simulink model "Electrical_System_2018b_obfs"  (R2019b)
settings: Solver=VariableStepAuto  StartTime=0.0  StopTime=5  RelTol=1e-3  AbsTol=1e-3  EnableMultiTasking=on
InitFcn:
  | Steady_State_Initialisation;
StopFcn:
  | %sscexplore(simlog);
  | %Logging
undefined symbols (not defined in the file): abrlhklxvp, aexgmhuedq, afmfmjnutg, afpphrjpnc, ahuxbyvruc, alarvljztt, amxnyqmnuw, aodrlwvqie, aolhmuplyq, aqpmguuqkg, auesgwirzl, aurophlnng, awamelrhru, ayfhvxflxn, azxkacuhqc, babszerikg, bawhdqanwq, bevoqecvei, bltjvqbchx, bmqsuewujl, bsmyqjfgnf, btvjbsmnve, bywgxqeadw, bziaduxaer, bzmcmdqocb, bzsvyvetat, ccsjnrbsih, cdvenygxwh, cedkrnslhx, cjheorclzs, cjrdshrtqx, ckhavyhcza, ckxewznhlz, cmrcgyiplk, conenicnws, cqkejbgjnn, csfnuwymhe, cunupkhwbh, cwzfvzuxxh, dcadmadufn, dcfponivnv, ddtrqjrhjn, dfhoxvkqas, dfrhtcwpne, dfvomcagjv, djijwylxea, dnmeqksrrm, dnzewbdkaa, dsqcykyxav, dtswwlttmm, ecumpidjtv, edegaywrct, ejjjsmnejc, eknqnehjdz, emvdetzouf, esxbqkbahr, etnkkbreiq, eunoiiiirw, ewewcuedir, fatkfxdhtc ... (+386)
libraries: fl_lib x802, ee_lib x362, fl_ps_legacy_lib x160, nesl_utility x85
(part 11 of 26)

== system Electrical_System_2018b_obfs/Redacted_1221/Redacted_7996/Redacted_1/Redacted_4377/Redacted_6082/Redacted_4288 ==
  Redacted_1420 : ee_lib/Passive/Thermal/Thermal Resistor  R=csfnuwymhe K/W  T_specify=off  T_priority=None  T=dfrhtcwpne K  T_nominal_specify=off  T_nominal_unit=K  T_nominal_value=undcbzrngw  Q_specify=off  Q_priority=None  Q=qyyvrynvtf W  Q_nominal_specify=off  Q_nominal_unit=W  Q_nominal_value=fykywgxewt
      settings: SourceProductName=Simscape Electrical  SourceProductBaseCode=PS  InternalSimscapePortConfiguration="{\"Bottom\":[],\"Left\":[{\"id\":\"A\",\"label\":\"A\",\"type\":\"foundation.thermal.thermal\"}],\"Right\":[{\"id\":\"B\",\"label\":\"B\",\"type\":\"foundation.thermal.thermal\"}],\"Top\":[]}"
  Redacted_3053 : ee_lib/Passive/Thermal/Thermal Resistor  R=feuklzgtpa K/W  T_specify=off  T_priority=None  T=qwktvjvfys K  T_nominal_specify=off  T_nominal_unit=K  T_nominal_value=arolkdlhmd  Q_specify=off  Q_priority=None  Q=djhelqxest W  Q_nominal_specify=off  Q_nominal_unit=W  Q_nominal_value=dkqmeratgj
      settings: SourceProductName=Simscape Electrical  SourceProductBaseCode=PS  InternalSimscapePortConfiguration="{\"Bottom\":[],\"Left\":[{\"id\":\"A\",\"label\":\"A\",\"type\":\"foundation.thermal.thermal\"}],\"Right\":[{\"id\":\"B\",\"label\":\"B\",\"type\":\"foundation.thermal.thermal\"}],\"Top\":[]}"
  Redacted_5187 : fl_lib/Electrical/Electrical Elements/Switch  R_closed=iidrcmgruo Ohm  G_open=cwflxapbrg 1/Ohm  Threshold=wtaszsnldr  i_specify=off  i_priority=None  i=cfjwrmlajq A  i_nominal_specify=off  i_nominal_unit=A  i_nominal_value=qzidrdxbsm  v_specify=off  v_priority=None  v=hrbzqwpexo V  v_nominal_specify=off  v_nominal_unit=V  v_nominal_value=oarcvjnccc
      settings: SourceProductName=Simscape
  Redacted_5716 : fl_lib/Electrical/Electrical Elements/Switch  R_closed=krkbgwsxlo Ohm  G_open=nwjalbnmwo 1/Ohm  Threshold=wlnjmfizfx  i_specify=off  i_priority=None  i=xtkvqzsayg A  i_nominal_specify=off  i_nominal_unit=A  i_nominal_value=nzimhpxyaj  v_specify=off  v_priority=None  v=dcozybqfae V  v_nominal_specify=off  v_nominal_unit=V  v_nominal_value=cwsubwwopk
      settings: SourceProductName=Simscape
  Redacted_631 : ee_lib/Semiconductors & Converters/Diode  ModelType=kwymznercn  Vf=bzeobnkmpp V  Ron=ogzcuqezum Ohm  Goff=hboakganul S  prmExp=tspwxvmtix  I12=vzhmfidnsx A  V12=lzcdoaedsk V  IS=lxuhqgdzyf A  ec=lgmvvpmtfb  I1=wubgixerlf A  V1=ghqnutyshn V  RS=yfueffmaxl Ohm  Tmeas=ydajfmxqbx degC  N_series=yivbhcvoir  N_parallel=htzntkphxa  Rz=qvvvhxwbpi Ohm  BV=ymjzdmieqs V  C_param=msvgljfcfw  CJ=zsrrieohii pF  CJ0=tuthjrqdnh pF  VJ=nycerhqgyj V  Mgrad=qvizemveid  Vvec=qlenbgnmqk V  Cvec=bligwbbtgp pF  FC=roozurrocc  Q_param=xkglsmbrbh  iRM=qahgubavsm A  iF=pufyexdedl A  didt=isjydruslg A/us  trr_factor=dffqwpsdyp  trr=anfkerbzue ns  Qrr=deomtvnwwe s*uA  TT=lrekwszonl ns  tau=iyastrgkxi ns  T_param=kjwuhembzs  IS_T2=mmckjlxiwy A  I1_T2=llsygjllnm A  V1_T2=ebzpqvnskm V  Tmeas2=dgihdwdint degC  EG_param=vfglbqzjmq  EG=vnjpxdvxmw eV  XTI_param=uocmdbuhnh  XTI=mybmalgdic  dBVdT=fpdhcmbsix V/K  Tdevice=fyegxrufcw degC  i_specify=off  i_priority=None  i=lkokslneyy A  i_nominal_specify=off  i_nominal_unit=A  i_nominal_value=hoeahmmfuu  v_specify=off  v_priority=None  v=jwstxjltpj V  v_nominal_specify=off  v_nominal_unit=V  v_nominal_value=vzfhxnllbc  i_capacitor_specify=off  i_capacitor_priority=None  i_capacitor=myvfxzqlck A  i_capacitor_nominal_specify=off  i_capacitor_nominal_unit=A  i_capacitor_nominal_value=roqvolylnm  v_capacitor_specify=off  v_capacitor_priority=None  v_capacitor=gptluhsrhz V  v_capacitor_nominal_specify=off  v_capacitor_nominal_unit=V  v_capacitor_nominal_value=alzbeepcwm  power_dissipated_specify=off  power_dissipated_priority=None  power_dissipated=uijibnuhos W  power_dissipated_nominal_specify=off  power_dissipated_nominal_unit=W  power_dissipated_nominal_value=lbddeeurpg  thermal_network_parameterization=frunhdzzzq  Rth=ipffswvaig K/W  Rth_Foster=tpgcjeuyzq K/W  thermal_mass_parameterization=jwlodfpkvm  thermal_mass=ehnyrrnqzl J/K  thermal_mass_Foster=unmbisyvtm J/K  thermal_time_constant=oypiywoukf s  thermal_time_constant_Foster=xnmvgxpcww s  thermal_mass_initial_temperatures=zwgjhousxc degC
      settings: SourceProductName=Simscape Electrical  InternalSimscapePortConfiguration="{\"Bottom\":[],\"Left\":[{\"id\":\"p\",\"label\":\"\",\"type\":\"foundation.electrical.electrical\"},{\"id\":\"H\",\"label\":\"H\",\"type\":\"foundation.thermal.thermal\"}],\"Right\":[{\"id\":\"n\",\"label\":\"\",\"type\":\"foundation.electrical.electrical\"}],\"Top\":[]}"
  Redacted_6763 : ee_lib/Semiconductors & Converters/Diode  ModelType=clgixcnwoc  Vf=ftpzcjmppy V  Ron=dbcidwevvn Ohm  Goff=yhrmcwzgue S  prmExp=aisizesfzq  I12=lacnnvocyc A  V12=pbpbsjubgs V  IS=xamdbquppu A  ec=eeecjfdprz  I1=yjljdcozpv A  V1=ffbopghzjw V  RS=wcqnbvzzev Ohm  Tmeas=kbuiibngbo degC  N_series=qqlilfwukw  N_parallel=fxbsiddyro  Rz=dodwndnmkr Ohm  BV=liehghwjmv V  C_param=vktsvahwle  CJ=fhntaxxfft pF  CJ0=qumaznckyu pF  VJ=xpoblmifuo V  Mgrad=ocusdggsnv  Vvec=seffqhedpz V  Cvec=ohcmggolrz pF  FC=yxsxrkinug  Q_param=bvzohlmuww  iRM=xicczpmsfr A  iF=rkcnntyhvb A  didt=vtudfiaipt A/us  trr_factor=rqvaooxfvk  trr=tvwihwyihb ns  Qrr=kulozvhoez s*uA  TT=nitkbtqglp ns  tau=ubqxhynwqh ns  T_param=igxsyorppi  IS_T2=mqvbxmpxvg A  I1_T2=armqecybmn A  V1_T2=muvfioogix V  Tmeas2=ppsjgixytg degC  EG_param=xjxvdcpxwh  EG=agihhvisij eV  XTI_param=yuocwdmjkw  XTI=xoszctygzp  dBVdT=uoohrvaigf V/K  Tdevice=qhfnbogqqg degC  i_specify=off  i_priority=None  i=qtedmgmqsm A  i_nominal_specify=off  i_nominal_unit=A  i_nominal_value=mqkthilpvy  v_specify=off  v_priority=None  v=itpbbundcp V  v_nominal_specify=off  v_nominal_unit=V  v_nominal_value=ykhzflpcnx  i_capacitor_specify=off  i_capacitor_priority=None  i_capacitor=uryfeeajta A  i_capacitor_nominal_specify=off  i_capacitor_nominal_unit=A  i_capacitor_nominal_value=ftxeerromd  v_capacitor_specify=off  v_capacitor_priority=None  v_capacitor=hddhodbyvb V  v_capacitor_nominal_specify=off  v_capacitor_nominal_unit=V  v_capacitor_nominal_value=yzdcvmjrfh  power_dissipated_specify=off  power_dissipated_priority=None  power_dissipated=aaxygncreu W  power_dissipated_nominal_specify=off  power_dissipated_nominal_unit=W  power_dissipated_nominal_value=xuxnetzqve  thermal_network_parameterization=zrkkuhurzb  Rth=odsbqwesbo K/W  Rth_Foster=ibbukupzba K/W  thermal_mass_parameterization=laqxzbiuja  thermal_mass=jqetfysksy J/K  thermal_mass_Foster=rleuvpzybd J/K  thermal_time_constant=vfwhldlplc s  thermal_time_constant_Foster=sredobdxmn s  thermal_mass_initial_temperatures=gkskoiqoer degC
      settings: SourceProductName=Simscape Electrical  InternalSimscapePortConfiguration="{\"Bottom\":[],\"Left\":[{\"id\":\"p\",\"label\":\"\",\"type\":\"foundation.electrical.electrical\"},{\"id\":\"H\",\"label\":\"H\",\"type\":\"foundation.thermal.thermal\"}],\"Right\":[{\"id\":\"n\",\"label\":\"\",\"type\":\"foundation.electrical.electrical\"}],\"Top\":[]}"
  Redacted_938 : ee_lib/Passive/Thermal/Thermal Resistor  R=virfgdrnfz K/W  T_specify=off  T_priority=None  T=alarvljztt K  T_nominal_specify=off  T_nominal_unit=K  T_nominal_value=joqgdgroxe  Q_specify=off  Q_priority=None  Q=kaqfzywiqi W  Q_nominal_specify=off  Q_nominal_unit=W  Q_nominal_value=zlmidgadwg
      settings: SourceProductName=Simscape Electrical  SourceProductBaseCode=PS  InternalSimscapePortConfiguration="{\"Bottom\":[],\"Left\":[{\"id\":\"A\",\"label\":\"A\",\"type\":\"foundation.thermal.thermal\"}],\"Right\":[{\"id\":\"B\",\"label\":\"B\",\"type\":\"foundation.thermal.thermal\"}],\"Top\":[]}"
  Redacted_2382 : PMIOPort  Side=Left
  Redacted_435 : PMIOPort  Port=2  Side=Left
  Redacted_3794 : PMIOPort  Port=3  Side=Right
  Redacted_28 : PMIOPort  Port=4  Side=Right
  Redacted_1383 : PMIOPort  Port=5  Side=Left
  Redacted_1778 : PMIOPort  Port=6  Side=Right
  connections:
  Redacted_6763/LConn1 -- Redacted_435/RConn1
  Redacted_6763/RConn1 -- Redacted_5716/LConn1
  Redacted_631/LConn2 -- Redacted_938/LConn1
  Redacted_3794/RConn1 -- Redacted_5187/RConn2
  Redacted_631/LConn1 -- Redacted_5187/LConn1
  Redacted_2382/RConn1 -- Redacted_631/RConn1
  Redacted_3053/RConn1 -- Redacted_1420/LConn1 -- Redacted_938/RConn1
  Redacted_1778/RConn1 -- Redacted_5716/RConn1 -- Redacted_5187/RConn1
  Redacted_28/RConn1 -- Redacted_5716/RConn2
  Redacted_1420/RConn1 -- Redacted_1383/RConn1
  Redacted_6763/LConn2 -- Redacted_3053/LConn1

== system Electrical_System_2018b_obfs/Redacted_1221/Redacted_7996/Redacted_1/Redacted_4377/Redacted_6082/Redacted_4413 ==
  Neutral_Negative : Subsystem  VariantControl=Variant1
  Positive_Neutral : Subsystem  VariantControl=Variant3
  Redacted_6190 : Subsystem  VariantControl=Variant2
  Redacted_9976 : PMIOPort  Side=Left
  Redacted_5180 : PMIOPort  Port=2  Side=Left
  Redacted_6712 : PMIOPort  Port=3  Side=Left
  Redacted_6595 : PMIOPort  Port=4  Side=Right
  Redacted_8408 : PMIOPort  Port=5  Side=Right

== system Electrical_System_2018b_obfs/Redacted_1221/Redacted_7996/Redacted_1/Redacted_4377/Redacted_6082/Redacted_4712 ==
  Redacted_2183 : ee_lib/Passive/Thermal/Thermal Resistor  R=uwrxzutslg K/W  T_specify=off  T_priority=None  T=pajgcmnuxp K  T_nominal_specify=off  T_nominal_unit=K  T_nominal_value=oprwgenfni  Q_specify=off  Q_priority=None  Q=vnctjcpbal W  Q_nominal_specify=off  Q_nominal_unit=W  Q_nominal_value=rnairkbzzr
      settings: SourceProductName=Simscape Electrical  SourceProductBaseCode=PS  InternalSimscapePortConfiguration="{\"Bottom\":[],\"Left\":[{\"id\":\"A\",\"label\":\"A\",\"type\":\"foundation.thermal.thermal\"}],\"Right\":[{\"id\":\"B\",\"label\":\"B\",\"type\":\"foundation.thermal.thermal\"}],\"Top\":[]}"
  Redacted_2562 : fl_lib/Electrical/Electrical Elements/Switch  R_closed=vkroixkmza Ohm  G_open=aclkmnqnqn 1/Ohm  Threshold=mqphwqpqtk  i_specify=off  i_priority=None  i=wqsnzdmaqu A  i_nominal_specify=off  i_nominal_unit=A  i_nominal_value=jdsbnyvvrn  v_specify=off  v_priority=None  v=mtgnvxvoef V  v_nominal_specify=off  v_nominal_unit=V  v_nominal_value=xpdcqtwjkq
      settings: SourceProductName=Simscape
  Redacted_4076 : fl_lib/Electrical/Electrical Elements/Switch  R_closed=njwxpudroe Ohm  G_open=unopnvzees 1/Ohm  Threshold=vnjqsgeems  i_specify=off  i_priority=None  i=tvyggmthfk A  i_nominal_specify=off  i_nominal_unit=A  i_nominal_value=fudhxnvthp  v_specify=off  v_priority=None  v=blecxtmuzk V  v_nominal_specify=off  v_nominal_unit=V  v_nominal_value=mxbomhtqdj
      settings: SourceProductName=Simscape
  Redacted_4934 : ee_lib/Passive/Thermal/Thermal Resistor  R=qtaxfrwwfd K/W  T_specify=off  T_priority=None  T=jbhnvsqxgq K  T_nominal_specify=off  T_nominal_unit=K  T_nominal_value=wqgbotzlrn  Q_specify=off  Q_priority=None  Q=oiubxlneqr W  Q_nominal_specify=off  Q_nominal_unit=W  Q_nominal_value=qhrxutyvpm
      settings: SourceProductName=Simscape Electrical  SourceProductBaseCode=PS  InternalSimscapePortConfiguration="{\"Bottom\":[],\"Left\":[{\"id\":\"A\",\"label\":\"A\",\"type\":\"foundation.thermal.thermal\"}],\"Right\":[{\"id\":\"B\",\"label\":\"B\",\"type\":\"foundation.thermal.thermal\"}],\"Top\":[]}"
  Redacted_6160 : ee_lib/Semiconductors & Converters/Diode  ModelType=wxghzbmewo  Vf=incyrzxxzf V  Ron=bufhejqsgj Ohm  Goff=bzmmwltpda S  prmExp=oyufyuxxul  I12=zqevqndhvr A  V12=ntgabtemlm V  IS=esogqbbpag A  ec=mhmrjglsyl  I1=baysikteys A  V1=jddnlczanv V  RS=xilzloxftw Ohm  Tmeas=hshgidoefp degC  N_series=tvwlqlappu  N_parallel=ynyhscmuqe  Rz=biacdhtehh Ohm  BV=vcztypyixs V  C_param=ymjusrygft  CJ=nzixmodzqw pF  CJ0=rmyzhcbopm pF  VJ=texbhuncud V  Mgrad=tkridumood  Vvec=jbuxjwgifj V  Cvec=yijsdqpcdn pF  FC=joqholwqmr  Q_param=iqextqebao  iRM=oosasuiphy A  iF=aqxfnvhdsh A  didt=iuypvkuhmr A/us  trr_factor=dqnmklrpvy  trr=rwbczlghkl ns  Qrr=ashruozjcw s*uA  TT=bxoqkmimcn ns  tau=upkecktgtn ns  T_param=whgrtbtgkt  IS_T2=ytmdinuaho A  I1_T2=poblvhcxkr A  V1_T2=hnwmatqgpq V  Tmeas2=jrgnekkvfk degC  EG_param=tblraoxtej  EG=timwdxryfu eV  XTI_param=btzoraanbl  XTI=wflfvuhjxp  dBVdT=xvknpvwxts V/K  Tdevice=gmzsticnnk degC  i_specify=off  i_priority=None  i=qefslitdry A  i_nominal_specify=off  i_nominal_unit=A  i_nominal_value=qcpugyhbqw  v_specify=off  v_priority=None  v=gggiokbjmg V  v_nominal_specify=off  v_nominal_unit=V  v_nominal_value=scytvwxumi  i_capacitor_specify=off  i_capacitor_priority=None  i_capacitor=qsjysvanbz A  i_capacitor_nominal_specify=off  i_capacitor_nominal_unit=A  i_capacitor_nominal_value=pewfqtvxxi  v_capacitor_specify=off  v_capacitor_priority=None  v_capacitor=bwoefqwwqs V  v_capacitor_nominal_specify=off  v_capacitor_nominal_unit=V  v_capacitor_nominal_value=mkonfywlen  power_dissipated_specify=off  power_dissipated_priority=None  power_dissipated=xgzyrlewkb W  power_dissipated_nominal_specify=off  power_dissipated_nominal_unit=W  power_dissipated_nominal_value=xaufgjttes  thermal_network_parameterization=rhtfzdpkld  Rth=aqkrjbornc K/W  Rth_Foster=cnqtfsutib K/W  thermal_mass_parameterization=xysbimjfwi  thermal_mass=ujjibidbol J/K  thermal_mass_Foster=dehixscchy J/K  thermal_time_constant=prtxkbhlrj s  thermal_time_constant_Foster=tazbjthomj s  thermal_mass_initial_temperatures=qkntalstxl degC
      settings: SourceProductName=Simscape Electrical  InternalSimscapePortConfiguration="{\"Bottom\":[],\"Left\":[{\"id\":\"p\",\"label\":\"\",\"type\":\"foundation.electrical.electrical\"},{\"id\":\"H\",\"label\":\"H\",\"type\":\"foundation.thermal.thermal\"}],\"Right\":[{\"id\":\"n\",\"label\":\"\",\"type\":\"foundation.electrical.electrical\"}],\"Top\":[]}"
  Redacted_7653 : ee_lib/Passive/Thermal/Thermal Resistor  R=tnulhwbazf K/W  T_specify=off  T_priority=None  T=mbqcmvdwox K  T_nominal_specify=off  T_nominal_unit=K  T_nominal_value=ayrbujabnr  Q_specify=off  Q_priority=None  Q=sfclfeggiu W  Q_nominal_specify=off  Q_nominal_unit=W  Q_nominal_value=pymdwgyhnk
      settings: SourceProductName=Simscape Electrical  SourceProductBaseCode=PS  InternalSimscapePortConfiguration="{\"Bottom\":[],\"Left\":[{\"id\":\"A\",\"label\":\"A\",\"type\":\"foundation.thermal.thermal\"}],\"Right\":[{\"id\":\"B\",\"label\":\"B\",\"type\":\"foundation.thermal.thermal\"}],\"Top\":[]}"
  Redacted_9027 : ee_lib/Semiconductors & Converters/Diode  ModelType=jyvxukpdpk  Vf=bdzbpjqkhz V  Ron=lsrjkjootd Ohm  Goff=ofmhtwesaf S  prmExp=bqtdjjwwji  I12=gwyojwxtvw A  V12=tjdwtiqjfm V  IS=pgunbsejse A  ec=gcomlckvkr  I1=iyetrhoopj A  V1=sdybwsehud V  RS=grqlbazvzm Ohm  Tmeas=ctncekrqyd degC  N_series=lxcnowzijw  N_parallel=kurybpjfoc  Rz=txvsbexxwk Ohm  BV=qqelmgxeqk V  C_param=zurgtvxcpf  CJ=nwcsymntkb pF  CJ0=qrfdvnulrv pF  VJ=mgmovfuewc V  Mgrad=ylqxslmpro  Vvec=afcdrhtwnp V  Cvec=gvbmqiulel pF  FC=xunkludvda  Q_param=kbqdjuiass  iRM=rpckqftvfb A  iF=sfeexggdhz A  didt=shdkxcjxfv A/us  trr_factor=jwvirxkxqn  trr=ftzljhgcnc ns  Qrr=upgxindely s*uA  TT=gisgyovfed ns  tau=oqxondjpzp ns  T_param=twxwcrqyec  IS_T2=yfadtlfwty A  I1_T2=yggssgboom A  V1_T2=utgekkynuc V  Tmeas2=osyodgdjlq degC  EG_param=qlkmxtofme  EG=idmsvcfrui eV  XTI_param=toxygxrvnh  XTI=iqhrhfuotd  dBVdT=rgeumoszgp V/K  Tdevice=ffqcgjdiix degC  i_specify=off  i_priority=None  i=bvvibiwhbr A  i_nominal_specify=off  i_nominal_unit=A  i_nominal_value=mnunjczkoc  v_specify=off  v_priority=None  v=zmmshkmtap V  v_nominal_specify=off  v_nominal_unit=V  v_nominal_value=sxmikghxbz  i_capacitor_specify=off  i_capacitor_priority=None  i_capacitor=hcljvkrkqs A  i_capacitor_nominal_specify=off  i_capacitor_nominal_unit=A  i_capacitor_nominal_value=csfodcmgpw  v_capacitor_specify=off  v_capacitor_priority=None  v_capacitor=lettjcqhzu V  v_capacitor_nominal_specify=off  v_capacitor_nominal_unit=V  v_capacitor_nominal_value=fmknydcgsh  power_dissipated_specify=off  power_dissipated_priority=None  power_dissipated=cmvyfkkapt W  power_dissipated_nominal_specify=off  power_dissipated_nominal_unit=W  power_dissipated_nominal_value=gwrobtedsy  thermal_network_parameterization=eykjzgpdvd  Rth=owkxttcwsg K/W  Rth_Foster=lhrazsinzy K/W  thermal_mass_parameterization=rnjojqvdyx  thermal_mass=omrqgtmzbh J/K  thermal_mass_Foster=agkrdtsffb J/K  thermal_time_constant=oqcaefzlvx s  thermal_time_constant_Foster=zpwspxdrsh s  thermal_mass_initial_temperatures=ksvqxybetb degC
      settings: SourceProductName=Simscape Electrical  InternalSimscapePortConfiguration="{\"Bottom\":[],\"Left\":[{\"id\":\"p\",\"label\":\"\",\"type\":\"foundation.electrical.electrical\"},{\"id\":\"H\",\"label\":\"H\",\"type\":\"foundation.thermal.thermal\"}],\"Right\":[{\"id\":\"n\",\"label\":\"\",\"type\":\"foundation.electrical.electrical\"}],\"Top\":[]}"
  Redacted_7604 : PMIOPort  Side=Left
  Redacted_7317 : PMIOPort  Port=2  Side=Left
  Redacted_2449 : PMIOPort  Port=3  Side=Right
  Redacted_1058 : PMIOPort  Port=4  Side=Right
  Redacted_1722 : PMIOPort  Port=5  Side=Left
  Redacted_8069 : PMIOPort  Port=6  Side=Right
  connections:
  Redacted_6160/LConn2 -- Redacted_4934/LConn1
  Redacted_7653/RConn1 -- Redacted_1722/RConn1
  Redacted_1058/RConn1 -- Redacted_2562/RConn2
  Redacted_4076/RConn1 -- Redacted_2562/RConn1 -- Redacted_8069/RConn1
  Redacted_2183/RConn1 -- Redacted_7653/LConn1 -- Redacted_4934/RConn1
  Redacted_7604/RConn1 -- Redacted_9027/RConn1
  Redacted_9027/LConn1 -- Redacted_4076/LConn1
  Redacted_2449/RConn1 -- Redacted_4076/RConn2
  Redacted_9027/LConn2 -- Redacted_2183/LConn1
  Redacted_6160/RConn1 -- Redacted_2562/LConn1
  Redacted_6160/LConn1 -- Redacted_7317/RConn1

== system Electrical_System_2018b_obfs/Redacted_1221/Redacted_7996/Redacted_1/Redacted_4377/Redacted_6082/Redacted_5129 ==
  Redacted_1091 : ee_lib/Passive/Thermal/Thermal Resistor  R=xukkryhjsj K/W  T_specify=off  T_priority=None  T=tqiwxmipjo K  T_nominal_specify=off  T_nominal_unit=K  T_nominal_value=aelkngfktz  Q_specify=off  Q_priority=None  Q=uecypvqdqw W  Q_nominal_specify=off  Q_nominal_unit=W  Q_nominal_value=dfxrifobdg
      settings: SourceProductName=Simscape Electrical  SourceProductBaseCode=PS  InternalSimscapePortConfiguration="{\"Bottom\":[],\"Left\":[{\"id\":\"A\",\"label\":\"A\",\"type\":\"foundation.thermal.thermal\"}],\"Right\":[{\"id\":\"B\",\"label\":\"B\",\"type\":\"foundation.thermal.thermal\"}],\"Top\":[]}"
  Redacted_3516 : fl_lib/Electrical/Electrical Elements/Switch  R_closed=viaptkjwzx Ohm  G_open=spahjfgthv 1/Ohm  Threshold=dnzewbdkaa  i_specify=off  i_priority=None  i=solngxsjde A  i_nominal_specify=off  i_nominal_unit=A  i_nominal_value=kcgnlcicvg  v_specify=off  v_priority=None  v=pvqprocfho V  v_nominal_specify=off  v_nominal_unit=V  v_nominal_value=hvyevfetqr
      settings: SourceProductName=Simscape
  Redacted_4493 : ee_lib/Passive/Thermal/Thermal Resistor  R=vkzgeqezuu K/W  T_specify=off  T_priority=None  T=esxbqkbahr K  T_nominal_specify=off  T_nominal_unit=K  T_nominal_value=kzpyjzolsz  Q_specify=off  Q_priority=None  Q=zidswjyook W  Q_nominal_specify=off  Q_nominal_unit=W  Q_nominal_value=mpaskulynn
      settings: SourceProductName=Simscape Electrical  SourceProductBaseCode=PS  InternalSimscapePortConfiguration="{\"Bottom\":[],\"Left\":[{\"id\":\"A\",\"label\":\"A\",\"type\":\"foundation.thermal.thermal\"}],\"Right\":[{\"id\":\"B\",\"label\":\"B\",\"type\":\"foundation.thermal.thermal\"}],\"Top\":[]}"
  Redacted_5736 : ee_lib/Semiconductors & Converters/Diode  ModelType=scnymfcyan  Vf=usjfqlowdb V  Ron=jptklmkxco Ohm  Goff=ihriznynzt S  prmExp=aymyrnkeyq  I12=sbueuqiyue A  V12=xralefmnmn V  IS=aazejvtdlh A  ec=lidbrydnsj  I1=aanjbxmvih A  V1=csezzhepis V  RS=hlsmvzlbct Ohm  Tmeas=qwpxhludyc degC  N_series=ngscuduecf  N_parallel=mtvctablcr  Rz=kfmndsfqah Ohm  BV=bisvtzzlmp V  C_param=zzuhuqdxbf  CJ=dgdyeqdnad pF  CJ0=vviixrlmuw pF  VJ=erikpjzwum V  Mgrad=idrwctvgka  Vvec=okvogmauev V  Cvec=ltbtlumqgo pF  FC=hutzvqbjst  Q_param=tfxaxdyfov  iRM=mxcantmjiz A  iF=xjldnwmowj A  didt=knlmkgueiv A/us  trr_factor=zjmxnibovs  trr=xbruedlduk ns  Qrr=rqbcaonvzx s*uA  TT=sescozsnne ns  tau=onhgnodkyy ns  T_param=plqnodbxtj  IS_T2=gunyrtbbui A  I1_T2=kbaugpgxig A  V1_T2=pfkhkcpzef V  Tmeas2=tqjznseuwe degC  EG_param=derhodxtrf  EG=puioajbhgt eV  XTI_param=kgeisxvirz  XTI=ttohkaatoo  dBVdT=qouasokgzj V/K  Tdevice=hapcaufila degC  i_specify=off  i_priority=None  i=fhzvmzekzz A  i_nominal_specify=off  i_nominal_unit=A  i_nominal_value=gxbmpayvch  v_specify=off  v_priority=None  v=busuwkvnmf V  v_nominal_specify=off  v_nominal_unit=V  v_nominal_value=mquxmvisyo  i_capacitor_specify=off  i_capacitor_priority=None  i_capacitor=erdhqvbuqo A  i_capacitor_nominal_specify=off  i_capacitor_nominal_unit=A  i_capacitor_nominal_value=rircubgbtn  v_capacitor_specify=off  v_capacitor_priority=None  v_capacitor=ivjksolhtz V  v_capacitor_nominal_specify=off  v_capacitor_nominal_unit=V  v_capacitor_nominal_value=fbdfrcucsm  power_dissipated_specify=off  power_dissipated_priority=None  power_dissipated=kcgakdxjwx W  power_dissipated_nominal_specify=off  power_dissipated_nominal_unit=W  power_dissipated_nominal_value=hmtdzvxlgr  thermal_network_parameterization=ahnuexnajx  Rth=zqvcvxpppv K/W  Rth_Foster=pikijtguhr K/W  thermal_mass_parameterization=ebiijoiwcx  thermal_mass=xdfmtdtgha J/K  thermal_mass_Foster=alrgsxgqtc J/K  thermal_time_constant=vinydwuarm s  thermal_time_constant_Foster=gzkwvsvsmy s  thermal_mass_initial_temperatures=fpaqdrttzj degC
      settings: SourceProductName=Simscape Electrical  InternalSimscapePortConfiguration="{\"Bottom\":[],\"Left\":[{\"id\":\"p\",\"label\":\"\",\"type\":\"foundation.electrical.electrical\"},{\"id\":\"H\",\"label\":\"H\",\"type\":\"foundation.thermal.thermal\"}],\"Right\":[{\"id\":\"n\",\"label\":\"\",\"type\":\"foundation.electrical.electrical\"}],\"Top\":[]}"
  Redacted_5773 : ee_lib/Passive/Thermal/Thermal Resistor  R=pbykuyqcdd K/W  T_specify=off  T_priority=None  T=wxiejlvzgg K  T_nominal_specify=off  T_nominal_unit=K  T_nominal_value=mfkuttxvwe  Q_specify=off  Q_priority=None  Q=dxpebethas W  Q_nominal_specify=off  Q_nominal_unit=W  Q_nominal_value=tsjrjrjwno
      settings: SourceProductName=Simscape Electrical  SourceProductBaseCode=PS  InternalSimscapePortConfiguration="{\"Bottom\":[],\"Left\":[{\"id\":\"A\",\"label\":\"A\",\"type\":\"foundation.thermal.thermal\"}],\"Right\":[{\"id\":\"B\",\"label\":\"B\",\"type\":\"foundation.thermal.thermal\"}],\"Top\":[]}"
  Redacted_7843 : ee_lib/Semiconductors & Converters/Diode  ModelType=vfubjonbyz  Vf=ovhazgcrzk V  Ron=cvrskrmuqj Ohm  Goff=lhhixvbmqc S  prmExp=qjndrrcrwj  I12=gntvzaamtj A  V12=wuwbzbrrpp V  IS=hzdxbkvqke A  ec=lzufgtgbsv  I1=zjffddejik A  V1=ijrimogulp V  RS=ykiqzyljzc Ohm  Tmeas=htzzchmtfv degC  N_series=hvcvcsiwkf  N_parallel=xydvemqmiv  Rz=otkhgvieqq Ohm  BV=vuygfstuny V  C_param=cqqyubkwai  CJ=uoegdangwr pF  CJ0=plaiwchowh pF  VJ=yenohlnnoo V  Mgrad=eruhhyqxpf  Vvec=svfoknpnpk V  Cvec=zqjlotgxpq pF  FC=ortnyuwzrh  Q_param=zdzueyncpy  iRM=pnzdzmfzlv A  iF=jwwiykcvrz A  didt=hhhqlcepyp A/us  trr_factor=rznizglpmy  trr=swvxsytfmb ns  Qrr=rqufmcdvlt s*uA  TT=pecnigvizl ns  tau=ijpnmgbmsc ns  T_param=qpvjlpxidl  IS_T2=vidgyzqclm A  I1_T2=khiphkkgwk A  V1_T2=pizjjevhmz V  Tmeas2=qreuemgwhd degC  EG_param=ancfqgfkip  EG=ktrhgbakxp eV  XTI_param=brbgadfkca  XTI=ygqbsywepo  dBVdT=eqvegiauyi V/K  Tdevice=drlcvrgbtu degC  i_specify=off  i_priority=None  i=cqcsuzhiqx A  i_nominal_specify=off  i_nominal_unit=A  i_nominal_value=xlakfqcnpk  v_specify=off  v_priority=None  v=hictgeopsi V  v_nominal_specify=off  v_nominal_unit=V  v_nominal_value=ughojcypmy  i_capacitor_specify=off  i_capacitor_priority=None  i_capacitor=hpzqydefid A  i_capacitor_nominal_specify=off  i_capacitor_nominal_unit=A  i_capacitor_nominal_value=tcfiupnxkj  v_capacitor_specify=off  v_capacitor_priority=None  v_capacitor=jmshvmneul V  v_capacitor_nominal_specify=off  v_capacitor_nominal_unit=V  v_capacitor_nominal_value=gayfmkqmju  power_dissipated_specify=off  power_dissipated_priority=None  power_dissipated=mgodbrjsas W  power_dissipated_nominal_specify=off  power_dissipated_nominal_unit=W  power_dissipated_nominal_value=fxyfgqyyze  thermal_network_parameterization=fvnzxsjdmp  Rth=wolwfjnjmr K/W  Rth_Foster=qclpxpisnk K/W  thermal_mass_parameterization=gxtwroopga  thermal_mass=inuccawayp J/K  thermal_mass_Foster=fypkvhimoq J/K  thermal_time_constant=rqyvbrsfkk s  thermal_time_constant_Foster=gsviadgrbu s  thermal_mass_initial_temperatures=udushfwxsp degC
      settings: SourceProductName=Simscape Electrical  InternalSimscapePortConfiguration="{\"Bottom\":[],\"Left\":[{\"id\":\"p\",\"label\":\"\",\"type\":\"foundation.electrical.electrical\"},{\"id\":\"H\",\"label\":\"H\",\"type\":\"foundation.thermal.thermal\"}],\"Right\":[{\"id\":\"n\",\"label\":\"\",\"type\":\"foundation.electrical.electrical\"}],\"Top\":[]}"
  Redacted_9825 : fl_lib/Electrical/Electrical Elements/Switch  R_closed=khogqsphcc Ohm  G_open=bnklxlqulg 1/Ohm  Threshold=bzmcmdqocb  i_specify=off  i_priority=None  i=debufxhmtc A  i_nominal_specify=off  i_nominal_unit=A  i_nominal_value=aobdrgvdef  v_specify=off  v_priority=None  v=jvrbptenmb V  v_nominal_specify=off  v_nominal_unit=V  v_nominal_value=ocwrndnqbv
      settings: SourceProductName=Simscape
  Redacted_3870 : PMIOPort  Side=Left
  Redacted_9209 : PMIOPort  Port=2  Side=Left
  Redacted_7831 : PMIOPort  Port=3  Side=Right
  Redacted_499 : PMIOPort  Port=4  Side=Right
  Redacted_8800 : PMIOPort  Port=5  Side=Left
  Redacted_5226 : PMIOPort  Port=6  Side=Right
  connections:
  Redacted_7843/LConn2 -- Redacted_5773/LConn1
  Redacted_4493/RConn1 -- Redacted_8800/RConn1
  Redacted_499/RConn1 -- Redacted_3516/RConn2
  Redacted_9825/RConn1 -- Redacted_3516/RConn1 -- Redacted_5226/RConn1
  Redacted_1091/RConn1 -- Redacted_4493/LConn1 -- Redacted_5773/RConn1
  Redacted_3870/RConn1 -- Redacted_5736/RConn1
  Redacted_5736/LConn1 -- Redacted_9825/LConn1
  Redacted_7831/RConn1 -- Redacted_9825/RConn2
  Redacted_5736/LConn2 -- Redacted_1091/LConn1
  Redacted_7843/RConn1 -- Redacted_3516/LConn1
  Redacted_7843/LConn1 -- Redacted_9209/RConn1

== system Electrical_System_2018b_obfs/Redacted_1221/Redacted_7996/Redacted_1/Redacted_4377/Redacted_6082/Redacted_538 ==
  Redacted_2474 : ee_lib/Passive/Thermal/Thermal Resistor  R=tlxbhmhcor K/W  T_specify=off  T_priority=None  T=glxcmexbqk K  T_nominal_specify=off  T_nominal_unit=K  T_nominal_value=rodxnpycsn  Q_specify=off  Q_priority=None  Q=qzyewlatml W  Q_nominal_specify=off  Q_nominal_unit=W  Q_nominal_value=gwgijjmpqo
      settings: SourceProductName=Simscape Electrical  SourceProductBaseCode=PS  InternalSimscapePortConfiguration="{\"Bottom\":[],\"Left\":[{\"id\":\"A\",\"label\":\"A\",\"type\":\"foundation.thermal.thermal\"}],\"Right\":[{\"id\":\"B\",\"label\":\"B\",\"type\":\"foundation.thermal.thermal\"}],\"Top\":[]}"
  Redacted_3959 : ee_lib/Semiconductors & Converters/Diode  ModelType=cvugfgmtfd  Vf=orelrxevia V  Ron=wxqqpmaddo Ohm  Goff=dngzjrqfwi S  prmExp=alwaagijeo  I12=ddqlkshwcb A  V12=xrkoiubeyy V  IS=xzqvhkoygc A  ec=mmbccpipxa  I1=ryagswhoik A  V1=yrovtgvtuv V  RS=cqohiqgcgo Ohm  Tmeas=hcgkqnpcsd degC  N_series=dhajyiyagh  N_parallel=twliypcbap  Rz=qwuyngymow Ohm  BV=nknpvrzxhu V  C_param=guvgzkombp  CJ=icairznadf pF  CJ0=mzqqqufhew pF  VJ=clgkkuemkj V  Mgrad=xeknterrpa  Vvec=epolkzdkro V  Cvec=ihzesxymmo pF  FC=renthmlyxq  Q_param=jdcgohbezp  iRM=qomoanohux A  iF=berhrdnhlf A  didt=nmtpqyoydb A/us  trr_factor=ellslhrnwb  trr=iwxktrkdlw ns  Qrr=lvsgqazssj s*uA  TT=djywuxkdvp ns  tau=dsvtaxiwkr ns  T_param=lkgbfzstdy  IS_T2=xxalayentz A  I1_T2=ouhmerbjva A  V1_T2=rsvjknjiop V  Tmeas2=gzwycyriyy degC  EG_param=ufydvnqgur  EG=awpclymgzc eV  XTI_param=hewsmdjtfl  XTI=uikenwfmwu  dBVdT=wnhlxqhthu V/K  Tdevice=oyhmqnvbqo degC  i_specify=off  i_priority=None  i=yuxtxukkqw A  i_nominal_specify=off  i_nominal_unit=A  i_nominal_value=tzdopizgpf  v_specify=off  v_priority=None  v=agbhwyzrpj V  v_nominal_specify=off  v_nominal_unit=V  v_nominal_value=ematotugcl  i_capacitor_specify=off  i_capacitor_priority=None  i_capacitor=xujmcaxirs A  i_capacitor_nominal_specify=off  i_capacitor_nominal_unit=A  i_capacitor_nominal_value=sdffyhujvl  v_capacitor_specify=off  v_capacitor_priority=None  v_capacitor=hxtlnoghbu V  v_capacitor_nominal_specify=off  v_capacitor_nominal_unit=V  v_capacitor_nominal_value=ulxhxpyrnl  power_dissipated_specify=off  power_dissipated_priority=None  power_dissipated=kejtoizjdb W  power_dissipated_nominal_specify=off  power_dissipated_nominal_unit=W  power_dissipated_nominal_value=zqnfawynfr  thermal_network_parameterization=drmprivida  Rth=ehoeehkluw K/W  Rth_Foster=rnfrlrqpxo K/W  thermal_mass_parameterization=qpxdavwohv  thermal_mass=dhvivgsoft J/K  thermal_mass_Foster=bbttosewnp J/K  thermal_time_constant=uruvbjugmy s  thermal_time_constant_Foster=vxxdggnndt s  thermal_mass_initial_temperatures=cxuqjhpxqo degC
      settings: SourceProductName=Simscape Electrical  InternalSimscapePortConfiguration="{\"Bottom\":[],\"Left\":[{\"id\":\"p\",\"label\":\"\",\"type\":\"foundation.electrical.electrical\"},{\"id\":\"H\",\"label\":\"H\",\"type\":\"foundation.thermal.thermal\"}],\"Right\":[{\"id\":\"n\",\"label\":\"\",\"type\":\"foundation.electrical.electrical\"}],\"Top\":[]}"
  Redacted_5204 : ee_lib/Semiconductors & Converters/Diode  ModelType=vhkfbcdxxi  Vf=hwocrhyzln V  Ron=nrejuoqraz Ohm  Goff=xoikkoxmpt S  prmExp=sshdgyqrid  I12=abapcaqksv A  V12=rcfonjwkhk V  IS=uxhycfgjjf A  ec=ccjnesusom  I1=dkqtptmenz A  V1=cwkuodtzyn V  RS=bilkvppmaj Ohm  Tmeas=yoefghiwnx degC  N_series=vbhwyhycfg  N_parallel=nkltgmwizt  Rz=hvsuszjqqa Ohm  BV=fiypzfmfcw V  C_param=oozhdefoba  CJ=sfgabkycgd pF  CJ0=fbfiajzyfi pF  VJ=oqefwzhbwp V  Mgrad=ljxgznyykq  Vvec=byqphrqwso V  Cvec=kiphagckdr pF  FC=cfchcpalde  Q_param=ctajamwbgf  iRM=zyzkgvwrwb A  iF=gzcqjdolru A  didt=ehosyigpsp A/us  trr_factor=yrcmqekjvi  trr=uxqgcepufe ns  Qrr=zdwkgjghcs s*uA  TT=gvqnwlgzwi ns  tau=vcapcgxzee ns  T_param=kdsbtpdywb  IS_T2=dytgzmkhng A  I1_T2=pmcdffsnwx A  V1_T2=yirsozpwmg V  Tmeas2=tadzfoaqtg degC  EG_param=lombnbdzaq  EG=syhamdjlbj eV  XTI_param=ujfmodxdji  XTI=pggidhagfw  dBVdT=jqycxgazic V/K  Tdevice=jamzfbwkuq degC  i_specify=off  i_priority=None  i=yrlsqtdcrj A  i_nominal_specify=off  i_nominal_unit=A  i_nominal_value=xvntcjckiw  v_specify=off  v_priority=None  v=jedxxskqdr V  v_nominal_specify=off  v_nominal_unit=V  v_nominal_value=havzscyyds  i_capacitor_specify=off  i_capacitor_priority=None  i_capacitor=tsjkkrkoym A  i_capacitor_nominal_specify=off  i_capacitor_nominal_unit=A  i_capacitor_nominal_value=gtnybtppoh  v_capacitor_specify=off  v_capacitor_priority=None  v_capacitor=kvzillyxwo V  v_capacitor_nominal_specify=off  v_capacitor_nominal_unit=V  v_capacitor_nominal_value=bigwvzuhqf  power_dissipated_specify=off  power_dissipated_priority=None  power_dissipated=hrgpyhajat W  power_dissipated_nominal_specify=off  power_dissipated_nominal_unit=W  power_dissipated_nominal_value=nzqvcegghq  thermal_network_parameterization=ptsabaosyw  Rth=gmkxekgtcr K/W  Rth_Foster=grktmnwzih K/W  thermal_mass_parameterization=bbnolzopgu  thermal_mass=mdlarzsjrd J/K  thermal_mass_Foster=bznhxpubkn J/K  thermal_time_constant=updbvvrtrk s  thermal_time_constant_Foster=thopflkoks s  thermal_mass_initial_temperatures=cwyiuwsawu degC
      settings: SourceProductName=Simscape Electrical  InternalSimscapePortConfiguration="{\"Bottom\":[],\"Left\":[{\"id\":\"p\",\"label\":\"\",\"type\":\"foundation.electrical.electrical\"},{\"id\":\"H\",\"label\":\"H\",\"type\":\"foundation.thermal.thermal\"}],\"Right\":[{\"id\":\"n\",\"label\":\"\",\"type\":\"foundation.electrical.electrical\"}],\"Top\":[]}"
  Redacted_5866 : ee_lib/Passive/Thermal/Thermal Resistor  R=yowuuinfal K/W  T_specify=off  T_priority=None  T=iyyjqewjxa K  T_nominal_specify=off  T_nominal_unit=K  T_nominal_value=cnwhogxdzi  Q_specify=off  Q_priority=None  Q=xatxitavcu W  Q_nominal_specify=off  Q_nominal_unit=W  Q_nominal_value=lovetezeec
      settings: SourceProductName=Simscape Electrical  SourceProductBaseCode=PS  InternalSimscapePortConfiguration="{\"Bottom\":[],\"Left\":[{\"id\":\"A\",\"label\":\"A\",\"type\":\"foundation.thermal.thermal\"}],\"Right\":[{\"id\":\"B\",\"label\":\"B\",\"type\":\"foundation.thermal.thermal\"}],\"Top\":[]}"
  Redacted_6815 : fl_lib/Electrical/Electrical Elements/Switch  R_closed=gkqjhdadlv Ohm  G_open=gspgtvvlfq 1/Ohm  Threshold=reaxmeylvl  i_specify=off  i_priority=None  i=jkwqanynmu A  i_nominal_specify=off  i_nominal_unit=A  i_nominal_value=retrrtohdd  v_specify=off  v_priority=None  v=bvhvmbtprm V  v_nominal_specify=off  v_nominal_unit=V  v_nominal_value=orfswznhsg
      settings: SourceProductName=Simscape
  Redacted_70 : ee_lib/Passive/Thermal/Thermal Resistor  R=radskbcesf K/W  T_specify=off  T_priority=None  T=pzbxgmpntj K  T_nominal_specify=off  T_nominal_unit=K  T_nominal_value=fxdfehzdjb  Q_specify=off  Q_priority=None  Q=wnpgpngqdb W  Q_nominal_specify=off  Q_nominal_unit=W  Q_nominal_value=mvvrjfvzjw
      settings: SourceProductName=Simscape Electrical  SourceProductBaseCode=PS  InternalSimscapePortConfiguration="{\"Bottom\":[],\"Left\":[{\"id\":\"A\",\"label\":\"A\",\"type\":\"foundation.thermal.thermal\"}],\"Right\":[{\"id\":\"B\",\"label\":\"B\",\"type\":\"foundation.thermal.thermal\"}],\"Top\":[]}"
  Redacted_8610 : fl_lib/Electrical/Electrical Elements/Switch  R_closed=ebbxigazsv Ohm  G_open=bymurvxztv 1/Ohm  Threshold=fatkfxdhtc  i_specify=off  i_priority=None  i=ooxbtdevdj A  i_nominal_specify=off  i_nominal_unit=A  i_nominal_value=vtutgwbqlf  v_specify=off  v_priority=None  v=bphxdwqdvi V  v_nominal_specify=off  v_nominal_unit=V  v_nominal_value=jxgusntfnc
      settings: SourceProductName=Simscape
  Redacted_1520 : PMIOPort  Side=Left
  Redacted_1920 : PMIOPort  Port=2  Side=Left
  Redacted_4965 : PMIOPort  Port=3  Side=Right
  Redacted_6828 : PMIOPort  Port=4  Side=Right
  Redacted_6082 : PMIOPort  Port=5  Side=Left
  Redacted_6905 : PMIOPort  Port=6  Side=Right
  connections:
  Redacted_3959/LConn1 -- Redacted_1920/RConn1
  Redacted_3959/RConn1 -- Redacted_6815/LConn1
  Redacted_5204/LConn2 -- Redacted_2474/LConn1
  Redacted_4965/RConn1 -- Redacted_8610/RConn2
  Redacted_5204/LConn1 -- Redacted_8610/LConn1
  Redacted_1520/RConn1 -- Redacted_5204/RConn1
  Redacted_5866/RConn1 -- Redacted_70/LConn1 -- Redacted_2474/RConn1
  Redacted_6905/RConn1 -- Redacted_6815/RConn1 -- Redacted_8610/RConn1
  Redacted_6828/RConn1 -- Redacted_6815/RConn2
  Redacted_70/RConn1 -- Redacted_6082/RConn1
  Redacted_3959/LConn2 -- Redacted_5866/LConn1

== system Electrical_System_2018b_obfs/Redacted_1221/Redacted_7996/Redacted_1/Redacted_4377/Redacted_6082/Redacted_5550 ==
  Neutral_Negative : Subsystem  VariantControl=Variant1
  Positive_Neutral : Subsystem  VariantControl=Variant3
  Redacted_2952 : Subsystem  VariantControl=Variant2
  Redacted_6826 : PMIOPort  Side=Left
  Redacted_51 : PMIOPort  Port=2  Side=Left
  Redacted_9515 : PMIOPort  Port=3  Side=Left
  Redacted_375 : PMIOPort  Port=4  Side=Right
  Redacted_6304 : PMIOPort  Port=5  Side=Right

== system Electrical_System_2018b_obfs/Redacted_1221/Redacted_7996/Redacted_1/Redacted_4377/Redacted_6082/Redacted_5711 ==
  Redacted_1131 : ee_lib/Semiconductors & Converters/Diode  ModelType=sgjcxllrwb  Vf=rezwarhnlc V  Ron=wbzpxlludr Ohm  Goff=tokjykannh S  prmExp=iwsikdclek  I12=ndxpqzjahu A  V12=oyqejwvxul V  IS=mveceiwvha A  ec=uuxcdrnxrh  I1=ofqmoxeuin A  V1=vhypwmzhjp V  RS=kpwjpdopvx Ohm  Tmeas=jbuqxwxids degC  N_series=xhtsnjlbqd  N_parallel=paajnctnwf  Rz=dwqreiwlqp Ohm  BV=yeooqkxzdk V  C_param=fuflydgeqt  CJ=ljpqbdycpo pF  CJ0=jbgrvpposm pF  VJ=ywlmgounuw V  Mgrad=zlqpkihwcd  Vvec=swnlxjsfea V  Cvec=tpransojiq pF  FC=teismtbows  Q_param=kzrgworrpy  iRM=enksfiblxd A  iF=bubyvkprkt A  didt=imidgzdgio A/us  trr_factor=kdehgjmswa  trr=ywtdexwfoq ns  Qrr=dyhowxpurl s*uA  TT=tdrpgsjpmg ns  tau=xwtxyhtqlh ns  T_param=kglbvnzolr  IS_T2=jjkoutammx A  I1_T2=hozxsnrmeo A  V1_T2=ojcyvtfvao V  Tmeas2=uzbilkqbml degC  EG_param=nqysccnfec  EG=ifucnavfam eV  XTI_param=wngxburzzp  XTI=ymmwmtduml  dBVdT=krekrcumku V/K  Tdevice=zrczwfcaxw degC  i_specify=off  i_priority=None  i=jssphwnvvg A  i_nominal_specify=off  i_nominal_unit=A  i_nominal_value=jibhoqemck  v_specify=off  v_priority=None  v=biwmugqnkj V  v_nominal_specify=off  v_nominal_unit=V  v_nominal_value=pllakottju  i_capacitor_specify=off  i_capacitor_priority=None  i_capacitor=gdasqvnftj A  i_capacitor_nominal_specify=off  i_capacitor_nominal_unit=A  i_capacitor_nominal_value=xlxqydjrzg  v_capacitor_specify=off  v_capacitor_priority=None  v_capacitor=jsbomwjeni V  v_capacitor_nominal_specify=off  v_capacitor_nominal_unit=V  v_capacitor_nominal_value=lbbdaqqoij  power_dissipated_specify=off  power_dissipated_priority=None  power_dissipated=ttqksqojpg W  power_dissipated_nominal_specify=off  power_dissipated_nominal_unit=W  power_dissipated_nominal_value=pktukgibmd  thermal_network_parameterization=ukdumittgs  Rth=xarbpsrvuf K/W  Rth_Foster=ehmdrospka K/W  thermal_mass_parameterization=igbepyqptu  thermal_mass=gcqxbhpikq J/K  thermal_mass_Foster=lennybeyrl J/K  thermal_time_constant=cyjedarpes s  thermal_time_constant_Foster=aczvdslxpi s  thermal_mass_initial_temperatures=vndblrhnsn degC
      settings: SourceProductName=Simscape Electrical  InternalSimscapePortConfiguration="{\"Bottom\":[],\"Left\":[{\"id\":\"p\",\"label\":\"\",\"type\":\"foundation.electrical.electrical\"},{\"id\":\"H\",\"label\":\"H\",\"type\":\"foundation.thermal.thermal\"}],\"Right\":[{\"id\":\"n\",\"label\":\"\",\"type\":\"foundation.electrical.electrical\"}],\"Top\":[]}"
  Redacted_2394 : fl_lib/Electrical/Electrical Elements/Switch  R_closed=softcbgoyi Ohm  G_open=mrgmmagxyi 1/Ohm  Threshold=afmfmjnutg  i_specify=off  i_priority=None  i=lmpryftbna A  i_nominal_specify=off  i_nominal_unit=A  i_nominal_value=rlcndthfub  v_specify=off  v_priority=None  v=qfybfotxik V  v_nominal_specify=off  v_nominal_unit=V  v_nominal_value=zyqcuaregq
      settings: SourceProductName=Simscape
  Redacted_3905 : ee_lib/Semiconductors & Converters/Diode  ModelType=nfeveyyrwk  Vf=zoxnipqvrl V  Ron=mtrtbspsae Ohm  Goff=dzrkkqnoys S  prmExp=ievifbrmqp  I12=mmnqlsbltn A  V12=iccotdqbos V  IS=mdvbhccktk A  ec=zvzvjmlaaq  I1=glkqrotric A  V1=yvlqfpnpng V  RS=nzwdscfish Ohm  Tmeas=nqkxyaekrd degC  N_series=nxssfyoknr  N_parallel=bahtqbhcpk  Rz=uddicyycvc Ohm  BV=lpfvklzlry V  C_param=fdmpjfrzqu  CJ=tlkmtlddns pF  CJ0=zlulxxuqkq pF  VJ=ehkmpglgid V  Mgrad=ttbwvlbyhc  Vvec=gsdwthuyom V  Cvec=lrvhhiuttc pF  FC=xzutmjviug  Q_param=qknxtjwyrl  iRM=prfitvseyr A  iF=kpkaitodiu A  didt=atkwyawqox A/us  trr_factor=utxssuipxd  trr=rrnoyzonvo ns  Qrr=dlavsnbofe s*uA  TT=ueprzvgvki ns  tau=jjxthajxlq ns  T_param=iixgioxeoz  IS_T2=wkxqlaxaiv A  I1_T2=zwqouuyrqp A  V1_T2=icvdtwdbib V  Tmeas2=quufchgzgc degC  EG_param=dwtsnaxksr  EG=acnxomkusk eV  XTI_param=vbeyylysip  XTI=xalaivvcmy  dBVdT=kxhlpasngh V/K  Tdevice=gzzizoikgr degC  i_specify=off  i_priority=None  i=tynowkxmpx A  i_nominal_specify=off  i_nominal_unit=A  i_nominal_value=uaygorgksr  v_specify=off  v_priority=None  v=tmrxmeyjrs V  v_nominal_specify=off  v_nominal_unit=V  v_nominal_value=bqcnnfwvrh  i_capacitor_specify=off  i_capacitor_priority=None  i_capacitor=imvbpaeqss A  i_capacitor_nominal_specify=off  i_capacitor_nominal_unit=A  i_capacitor_nominal_value=gybwnvfkmn  v_capacitor_specify=off  v_capacitor_priority=None  v_capacitor=igyzppqxtw V  v_capacitor_nominal_specify=off  v_capacitor_nominal_unit=V  v_capacitor_nominal_value=larocdhkvv  power_dissipated_specify=off  power_dissipated_priority=None  power_dissipated=lnzqmvpzim W  power_dissipated_nominal_specify=off  power_dissipated_nominal_unit=W  power_dissipated_nominal_value=spywrtkhsd  thermal_network_parameterization=hddxfofeyy  Rth=jullxwctpz K/W  Rth_Foster=nvhdmofkhg K/W  thermal_mass_parameterization=mkeqkoxjsc  thermal_mass=sxbbhkgscj J/K  thermal_mass_Foster=ktkpfefkzp J/K  thermal_time_constant=rzzrohaxsq s  thermal_time_constant_Foster=kpaqylfjiw s  thermal_mass_initial_temperatures=jazsdptkag degC
      settings: SourceProductName=Simscape Electrical  InternalSimscapePortConfiguration="{\"Bottom\":[],\"Left\":[{\"id\":\"p\",\"label\":\"\",\"type\":\"foundation.electrical.electrical\"},{\"id\":\"H\",\"label\":\"H\",\"type\":\"foundation.thermal.thermal\"}],\"Right\":[{\"id\":\"n\",\"label\":\"\",\"type\":\"foundation.electrical.electrical\"}],\"Top\":[]}"
  Redacted_5143 : ee_lib/Passive/Thermal/Thermal Resistor  R=ybijqqbkuj K/W  T_specify=off  T_priority=None  T=fxspchliwh K  T_nominal_specify=off  T_nominal_unit=K  T_nominal_value=ppuzbfrerj  Q_specify=off  Q_priority=None  Q=bynsukdflj W  Q_nominal_specify=off  Q_nominal_unit=W  Q_nominal_value=wzgdmbkzup
      settings: SourceProductName=Simscape Electrical  SourceProductBaseCode=PS  InternalSimscapePortConfiguration="{\"Bottom\":[],\"Left\":[{\"id\":\"A\",\"label\":\"A\",\"type\":\"foundation.thermal.thermal\"}],\"Right\":[{\"id\":\"B\",\"label\":\"B\",\"type\":\"foundation.thermal.thermal\"}],\"Top\":[]}"
  Redacted_5618 : fl_lib/Electrical/Electrical Elements/Switch  R_closed=kezykkwcel Ohm  G_open=kohltqvzvt 1/Ohm  Threshold=cdvenygxwh  i_specify=off  i_priority=None  i=hmjtisnfth A  i_nominal_specify=off  i_nominal_unit=A  i_nominal_value=nehnrbwlwu  v_specify=off  v_priority=None  v=yztjetatcm V  v_nominal_specify=off  v_nominal_unit=V  v_nominal_value=mbyxixcoyh
      settings: SourceProductName=Simscape
  Redacted_8133 : ee_lib/Passive/Thermal/Thermal Resistor  R=jumrqxyemk K/W  T_specify=off  T_priority=None  T=ohgunjtfhv K  T_nominal_specify=off  T_nominal_unit=K  T_nominal_value=iyidfkkalr  Q_specify=off  Q_priority=None  Q=paihpxggkf W  Q_nominal_specify=off  Q_nominal_unit=W  Q_nominal_value=epallypmhw
      settings: SourceProductName=Simscape Electrical  SourceProductBaseCode=PS  InternalSimscapePortConfiguration="{\"Bottom\":[],\"Left\":[{\"id\":\"A\",\"label\":\"A\",\"type\":\"foundation.thermal.thermal\"}],\"Right\":[{\"id\":\"B\",\"label\":\"B\",\"type\":\"foundation.thermal.thermal\"}],\"Top\":[]}"
  Redacted_9572 : ee_lib/Passive/Thermal/Thermal Resistor  R=ttoaasuswm K/W  T_specify=off  T_priority=None  T=nnfmlqeyqa K  T_nominal_specify=off  T_nominal_unit=K  T_nominal_value=fhorypsrxc  Q_specify=off  Q_priority=None  Q=ckuzftrrgq W  Q_nominal_specify=off  Q_nominal_unit=W  Q_nominal_value=fqmdqwvrwk
      settings: SourceProductName=Simscape Electrical  SourceProductBaseCode=PS  InternalSimscapePortConfiguration="{\"Bottom\":[],\"Left\":[{\"id\":\"A\",\"label\":\"A\",\"type\":\"foundation.thermal.thermal\"}],\"Right\":[{\"id\":\"B\",\"label\":\"B\",\"type\":\"foundation.thermal.thermal\"}],\"Top\":[]}"
  Redacted_4950 : PMIOPort  Side=Left
  Redacted_5258 : PMIOPort  Port=2  Side=Left
  Redacted_5892 : PMIOPort  Port=3  Side=Right
  Redacted_8207 : PMIOPort  Port=4  Side=Right
  Redacted_4180 : PMIOPort  Port=5  Side=Left
  Redacted_8951 : PMIOPort  Port=6  Side=Right
  connections:
  Redacted_3905/LConn2 -- Redacted_8133/LConn1
  Redacted_9572/RConn1 -- Redacted_4180/RConn1
  Redacted_8207/RConn1 -- Redacted_2394/RConn2
  Redacted_5618/RConn1 -- Redacted_2394/RConn1 -- Redacted_8951/RConn1
  Redacted_5143/RConn1 -- Redacted_9572/LConn1 -- Redacted_8133/RConn1
  Redacted_4950/RConn1 -- Redacted_1131/RConn1
  Redacted_1131/LConn1 -- Redacted_5618/LConn1
  Redacted_5892/RConn1 -- Redacted_5618/RConn2
  Redacted_1131/LConn2 -- Redacted_5143/LConn1
  Redacted_3905/RConn1 -- Redacted_2394/LConn1
  Redacted_3905/LConn1 -- Redacted_5258/RConn1

== system Electrical_System_2018b_obfs/Redacted_1221/Redacted_7996/Redacted_1/Redacted_4377/Redacted_6082/Redacted_5713 ==
  Neutral_Negative : Subsystem  VariantControl=Variant1
  Positive_Neutral : Subsystem  VariantControl=Variant3
  Redacted_1184 : Subsystem  VariantControl=Variant2
  Redacted_6138 : PMIOPort  Side=Left
  Redacted_1431 : PMIOPort  Port=2  Side=Left
  Redacted_7946 : PMIOPort  Port=3  Side=Left
  Redacted_819 : PMIOPort  Port=4  Side=Right
  Redacted_4816 : PMIOPort  Port=5  Side=Right

== system Electrical_System_2018b_obfs/Redacted_1221/Redacted_7996/Redacted_1/Redacted_4377/Redacted_6082/Redacted_5976 ==
  Neutral_Negative : Subsystem  VariantControl=Variant1
  Positive_Neutral : Subsystem  VariantControl=Variant3
  Redacted_5620 : Subsystem  VariantControl=Variant2
  Redacted_9241 : PMIOPort  Side=Left
  Redacted_5276 : PMIOPort  Port=2  Side=Left
  Redacted_2400 : PMIOPort  Port=3  Side=Left
  Redacted_5406 : PMIOPort  Port=4  Side=Right
  Redacted_1074 : PMIOPort  Port=5  Side=Right

== system Electrical_System_2018b_obfs/Redacted_1221/Redacted_7996/Redacted_1/Redacted_4377/Redacted_6082/Redacted_6424 ==
  Neutral_Negative : Subsystem  VariantControl=Variant1
  Positive_Neutral : Subsystem  VariantControl=Variant3
  Redacted_7805 : Subsystem  VariantControl=Variant2
  Redacted_4582 : PMIOPort  Side=Left
  Redacted_1544 : PMIOPort  Port=2  Side=Left
  Redacted_1581 : PMIOPort  Port=3  Side=Left
  Redacted_1961 : PMIOPort  Port=4  Side=Right
  Redacted_7479 : PMIOPort  Port=5  Side=Right
